simulink model "test_data"  (Simulink 8.6)
settings: Solver=FixedStepDiscrete  StartTime=0.0  StopTime=10.0  FixedStep=0.001  RelTol=1e-3
libraries: instrumentlib x2, simulink x1
settings Model: Creator=GIHOON  LastModifiedBy=GIHOON
settings DataIOCC: SaveFormat=Dataset  SignalLoggingSaveFormat=Dataset
settings OptimizationCC: ExpressionDepthLimit=128
settings DebuggingCC: UnderspecifiedInitializationDetection=Simplified  MergeDetectMultiDrivingBlocksExec=error  SolverPrmCheckMsg=none  FcnCallInpInsideContextMsg=EnableAllAsError  StateNameClashWarn=none
settings HardwareCC: ProdBitPerPointer=64  ProdLargestAtomicFloat=Float  ProdIntDivRoundTo=Zero  ProdEndianess=LittleEndian  ProdWordSize=64  ProdHWDeviceType=Intel->x86-64 (Windows64)
settings GRTTargetCC: GeneratePreprocessorConditionals=Use local settings  CombineOutputUpdateFcns=on  GRTInterface=off
settings ConfigComp: CovModelRefEnable=off

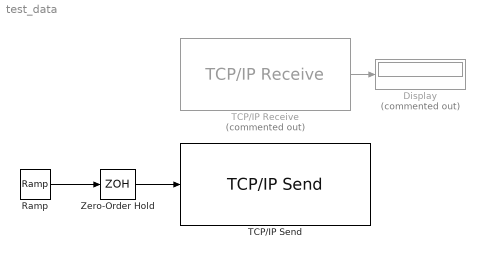
== system test_data ==
  Display : Display  Commented=on
  Ramp : simulink/Sources/Ramp  slope=1  start=1  X0=0
  TCP/IP Receive : instrumentlib/TCP//IP Receive  Commented=on  Host=localhost  Port=50007  DataSize=1  EnableBlockingMode=on  Timeout=10  SampleTime=0.001  DataType=double  ByteOrder=BigEndian
  TCP/IP Send : instrumentlib/TCP//IP Send  Host=localhost  Port=50007  EnableBlockingMode=on  Timeout=10  ByteOrder=BigEndian
  Zero-Order Hold : ZeroOrderHold  SampleTime=0.001
  wires:
  TCP/IP Receive/1 -> Display/1
  Ramp/1 -> Zero-Order Hold/1
  Zero-Order Hold/1 -> TCP/IP Send/1
